simulink model "Ssim3"  (Simulink 10.2)
settings: Solver=ode23  StartTime=0.0  StopTime=10  RelTol=1e-3  EnableMultiTasking=on
libraries: simulink x3
settings Model: Creator=hp  LastModifiedBy=11634
settings DataIOCC: LimitDataPoints=on  SignalLoggingName=sigsOut
settings OptimizationCC: ExpressionDepthLimit=2147483647  InitFltsAndDblsToZero=on
settings DebuggingCC: SaveWithParameterizedLinksMsg=none  SignalResolutionControl=TryResolveAllWithWarning  MultiTaskDSMMsg=warning  MultiTaskCondExecSysMsg=none  StateNameClashWarn=warning
settings HardwareCC: TargetUnknown=on
settings GRTTargetCC: TargetFcnLib=ansi_tfl_tmw.mat

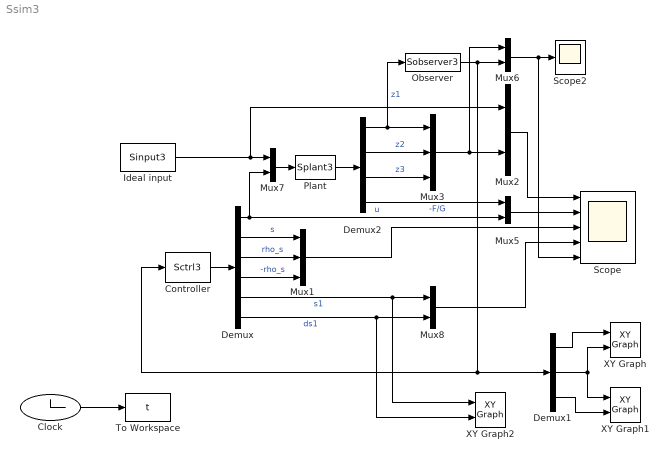
== system Ssim3 ==
  Clock : Clock
  Controller : S-Function  FunctionName=Sctrl3  SFunctionDeploymentMode=off  EnableBusSupport=off
  Demux : Demux  Outputs=6
  Demux1 : Demux  Outputs=3
  Demux2 : Demux
  Ideal input : S-Function  FunctionName=Sinput3  SFunctionDeploymentMode=off  EnableBusSupport=off
  Mux1 : Mux  Inputs=3
  Mux{2,5..8} (5 alike) : Mux  Inputs=2
  Mux3 : Mux  Inputs=3
  Observer : S-Function  FunctionName=Sobserver3  SFunctionDeploymentMode=off  EnableBusSupport=off
  Plant : S-Function  FunctionName=Splant3  SFunctionDeploymentMode=off  EnableBusSupport=off
  Scope : Scope  NumInputPorts=5
  Scope2 : Scope
  To Workspace : ToWorkspace  VariableName=t  SampleTime=-1
  XY Graph : simulink/Sinks/XY Graph  xmin=-1  xmax=2  ymin=-1  ymax=2  st=-1
  XY Graph1 : simulink/Sinks/XY Graph  xmin=-3  xmax=5  ymin=-6  ymax=2  st=-1
  XY Graph2 : simulink/Sinks/XY Graph  xmin=-5  xmax=3  ymin=-4  ymax=4  st=-1
  wires:
  Demux/1 -> Mux5/2, Mux7/2  "u"
  Clock/1 -> To Workspace/1
  Observer/1 -> Controller/1, Demux1/1, Mux6/2
  Ideal input/1 -> Mux2/1, Mux7/1
  Controller/1 -> Demux/1
  Demux1/1 -> XY Graph/1
  Demux1/2 -> XY Graph1/1, XY Graph/2
  Demux1/3 -> XY Graph1/2
  Mux2/1 -> Scope/1
  Demux/3 -> Mux1/2  "rho_s"
  Demux/2 -> Mux1/1  "s"
  Demux/4 -> Mux1/3  "-rho_s"
  Mux1/1 -> Scope/3
  Demux/5 -> XY Graph2/1, Mux8/1  "s1"
  Demux/6 -> XY Graph2/2, Mux8/2  "ds1"
  Demux2/2 -> Mux3/2  "z2"
  Demux2/1 -> Observer/1, Mux3/1  "z1"
  Demux2/3 -> Mux3/3  "z3"
  Plant/1 -> Demux2/1
  Demux2/4 -> Mux5/1  "-F/G"
  Mux5/1 -> Scope/2
  Mux3/1 -> Mux2/2, Mux6/1
  Mux6/1 -> Scope2/1, Scope/5
  Mux8/1 -> Scope/4
  Mux7/1 -> Plant/1
